simulink model "D_20231120_Modell_Inbetriebnahme_BreakOutBox_Jetson"  (R2022b)
settings: Solver=ode1  StartTime=0.0  StopTime=inf  FixedStep=Ts  RelTol=1e-3
PreLoadFcn:
  | pulsePeriod = 0.05;
  | 
  | Ts = 0.001;
  | 
  | FPGA_Frequency = 75000000;
  | 
  | ts_IO691 = 5e-3;
PostLoadFcn:
  | ewolfSetUp
InitFcn:
  | pulsePeriod = 0.05;
  | 
  | Ts = 0.001;
  | 
  | FPGA_Frequency = 75000000;
  | 
  | ts_IO691 = 5e-3;
StopFcn:
  | Simulink.sdi.clearPreferences;
  | if isfile(['sdi_view_',bdroot,'.mldatx'])
  | Simulink.sdi.view;
  | pause(3);
  | Simulink.sdi.loadView(['sdi_view_',bdroot,]);
  | end
model workspace (MAT data in the model file):
  MaxDreh = 1
values from neighbouring files (symbols this model uses):
  max_ac = 2    [ewolfSetUp.m]
  min_ac = -3    [ewolfSetUp.m]
  PredictionHorizon = 30    [ewolfSetUp.m]
undefined symbols (not defined in the file or in its folder): canChannel, DiscIntNeverNeededParam, Ended, HS, IO291, IO397, max_steer_car, min_steer_car, sigbuilder_block, Single
libraries: lllalib x255, canmsglib x146, simulink x42, speedgoatlib_IO191 x5, speedgoatlib_IO291 x5, slrealtimeiplib x3, speedgoatlib_IO691 x3, slrealtimeutilitieslib x2, spsEdgeDetectorLib x1, simulink_extras x1, speedgoatlib_fpga_dio x1, speedgoatlib_fpga_quadrature x1
(part 3 of 8)

== system D_20231120_Modell_Inbetriebnahme_BreakOutBox_Jetson/Freigabe/Freigabe/Detektion Lenkung ==
  note: Detektion Schwellwertüberschreitung (0,8)
  note: Dauer der Schwellwertüberschreitung > 0,2s?
  LG_1_In : Inport
  LG_2_In : Inport  Port=2
  Abs2 : Abs  SaturateOnIntegerOverflow=off
  Compare To Constant4 : simulink/Logic and Bit Operations/Compare To Constant  relop=>  const=0.8  OutDataTypeStr=boolean
  Data Type Conversion2 : DataTypeConversion  OutDataTypeStr=double  SaturateOnIntegerOverflow=off  RndMeth=Floor
  Delta_Time1 : Constant  Value=0.2
  Discrete-Time Integrator2 : DiscreteIntegrator  ExternalReset=falling  SampleTime=-1  ICPrevOutput=DiscIntNeverNeededParam  ICPrevScaledInput=DiscIntNeverNeededParam
  Relational Operator2 : RelationalOperator  Operator=<  OutDataTypeStr=boolean  RndMeth=Simplest  InputSameDT=off
  Subtract2 : Sum  Inputs=+-
  LG_Freigabe : Outport
  wires:
  LG_1_In/1 -> Subtract2/1
  LG_2_In/1 -> Subtract2/2
  Relational Operator2/1 -> LG_Freigabe/1
  Subtract2/1 -> Abs2/1
  Abs2/1 -> Compare To Constant4/1
  Data Type Conversion2/1 -> Discrete-Time Integrator2/2, Discrete-Time Integrator2/1
  Compare To Constant4/1 -> Data Type Conversion2/1
  Discrete-Time Integrator2/1 -> Relational Operator2/1
  Delta_Time1/1 -> Relational Operator2/2

== system D_20231120_Modell_Inbetriebnahme_BreakOutBox_Jetson/Freigabe/Freigabe/EMV Filter ==
  In : Inport
  Compare To Constant : simulink/Logic and Bit Operations/Compare To Constant  relop===  const=1  OutDataTypeStr=boolean
  Divide : Product  Inputs=*/
  Sum of Elements : Sum  Inputs=+
  Tapped Delay1 : simulink/Discrete/Tapped Delay  vinit=0.0  samptime=-1  NumDelays=4  DelayOrder=Oldest  includeCurrent=off
  Vector Concatenate : Concatenate
  Width : Width
  Out : Outport  VectorParamsAs1DForOutWhenUnconnected=off
  wires:
  In/1 -> Vector Concatenate/1, Tapped Delay1/1
  Tapped Delay1/1 -> Vector Concatenate/2
  Vector Concatenate/1 -> Sum of Elements/1, Width/1
  Divide/1 -> Compare To Constant/1
  Sum of Elements/1 -> Divide/1
  Width/1 -> Divide/2
  Compare To Constant/1 -> Out/1

== system D_20231120_Modell_Inbetriebnahme_BreakOutBox_Jetson/IO691/CAN Read Loop - Port 3/Enabled Subsystem ==
  CAN Msg : Inport
  Enable : EnablePort
  extract radar data from CAN msg stream : Subsystem  Description=|
      | Extract radar data from CAN messages and create vector object with: 1788 fields:
      | 
      | 1. Timestamp
      | 2. cycle_count
      | 3. number of Objects
      | 4. radar timestamp_header
      | 5. CAN ID
      | +++++++++++++++++++++
      | % last point
      | 6. range
      | 7. az
      | 8. vr
      | 9. rcs
      | 10. el
      | ----------------------------------
      | % last point -1
      | 11. range
      | 12. az
      | 13. vr
      | 14. rcs
      | 15. el
      |  ...
      | 
      | empty points, all values == 0
  enable outP : Outport
  data : Outport  Port=2
  Radar_Punkt : Outport  Port=3
  Radar_Mode : Outport  Port=4
  wires:
  CAN Msg/1 -> extract radar data from CAN msg stream/1(msg)
  extract radar data from CAN msg stream/1(enable outP) -> enable outP/1
  extract radar data from CAN msg stream/2(data) -> data/1
  extract radar data from CAN msg stream/3(Radar_Punkt) -> Radar_Punkt/1
  extract radar data from CAN msg stream/4(Radar_Mode) -> Radar_Mode/1

== system D_20231120_Modell_Inbetriebnahme_BreakOutBox_Jetson/IO691/CAN Read Loop - Port 3/Linearisierung Lenkwinkel IST ==
  Lenkradwinkel : Inport
  Divide : Product  Inputs=*/
  Ratio Lenkradwinkel Lenkwinkel : Constant  Value=20.3
  Lenkwinkel : Outport
  wires:
  Ratio Lenkradwinkel Lenkwinkel/1 -> Divide/2
  Divide/1 -> Lenkwinkel/1
  Lenkradwinkel/1 -> Divide/1
